simulink model "Plantilla_Simulink_Estanque"  (Simulink 8.1)
settings: Solver=ode5  StartTime=0.0  StopTime=5000  FixedStep=0.05  RelTol=1e-3
libraries: RT x1
settings Model: Creator=Alleon  LastModifiedBy=Admin
settings DataIOCC: LimitDataPoints=off  SaveOutput=off  SaveTime=off  SignalLoggingName=sigsOut
settings OptimizationCC: ExpressionDepthLimit=128  InitFltsAndDblsToZero=on
settings DebuggingCC: SaveWithParameterizedLinksMsg=none  SignalResolutionControl=TryResolveAllWithWarning  SolverPrmCheckMsg=none  MultiTaskDSMMsg=warning  MultiTaskCondExecSysMsg=none  StrictBusMsg=None
settings HardwareCC: TargetUnknown=on
settings SFSimCC: SimParseCustomCode=off
settings RTWCC: IncludeERTFirstTime=on
settings GRTTargetCC: TargetFcnLib=ansi_tfl_tmw.mat

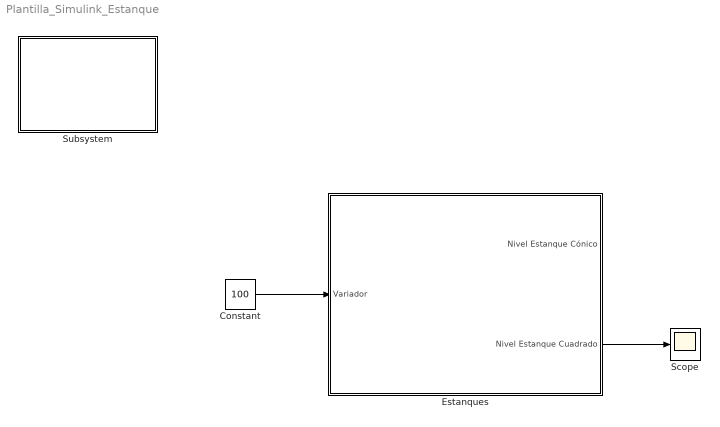
== system Plantilla_Simulink_Estanque ==
  Constant : Constant  Value=100
  Estanques : Subsystem  mask{D=off}
      mask prompts: D "Descarga"
      mask Display:
      | image(imread('img/estanque.png'))
      | 
      | port_label('input', 1, 'Variador')
      | port_label('output', 1, 'Nivel Estanque Conico')
      | port_label('output', 2, 'Nivel Estanque Cuadrado')
  Scope : Scope
      settings: TimeRange=5000  YMin=0  YMax=8.5
  Subsystem : Subsystem
      mask Display: image(imread('img/logo.png'))
  wires:
  Constant/1 -> Estanques/1("Variador ")
  Estanques/2("Nivel Estanque Cuadrado ") -> Scope/1

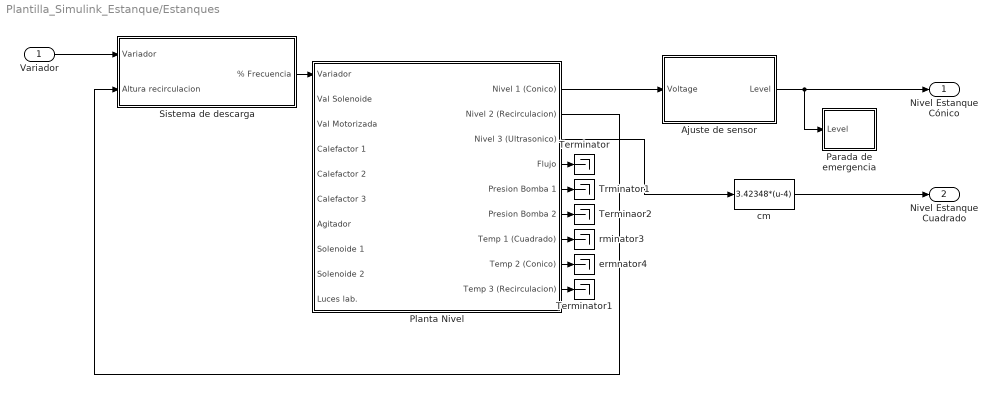
== system Plantilla_Simulink_Estanque/Estanques ==
  "Variador " : Inport
  Ajuste de sensor : Subsystem  mask(Ajuste de sensor){SE=6.53, SL=-0.1}
      mask prompts: SE "Correccion error de sensor"; SL "Limite inferior sensor"
      mask help: Calibra el sensor y transforma la señal de corriente en altura en cms.
  Parada de emergencia : Subsystem  mask(Parada de Emergencia){ML=65}
      mask prompts: ML "Umbral maximo altura"
      mask help: Define el umbral de altura para activar la parada de emergencia.
  Planta Nivel : Subsystem  mask{Ts=0.05}
      mask prompts: Ts "Tiempo Muestreo"
      mask help: Planta de Nivel
  Sistema de descarga : Subsystem  mask{SA=5.28, OT=0.25}
      mask prompts: SA "Ajuste de sensor"; OT "Umbral de apagado"
  Terminaor2 : Terminator
  Terminator : Terminator
  Terminator1 : Terminator
  Trminator1 : Terminator
  cm : Fcn  Expr=3.42348*(u-4)
  ermnator4 : Terminator
  rminator3 : Terminator
  Nivel Estanque Cónico : Outport
  "Nivel Estanque Cuadrado " : Outport  Port=2
  wires:
  Planta Nivel/1(Nivel 1 (Conico)) -> Ajuste de sensor/1(Voltage)
  Planta Nivel/3(Nivel 3 (Ultrasonico)) -> cm/1
  cm/1 -> "Nivel Estanque Cuadrado "/1
  "Variador "/1 -> Sistema de descarga/1(Variador)
  Ajuste de sensor/1(Level) -> Nivel Estanque Cónico/1, Parada de emergencia/1(Level)
  Planta Nivel/2(Nivel 2 (Recirculacion)) -> Sistema de descarga/2(Altura recirculacion)
  Sistema de descarga/1(% Frecuencia) -> Planta Nivel/1(Variador)
  Planta Nivel/4(Flujo) -> Terminator/1
  Planta Nivel/5(Presion Bomba 1) -> Trminator1/1
  Planta Nivel/6(Presion Bomba 2) -> Terminaor2/1
  Planta Nivel/7(Temp 1 (Cuadrado)) -> rminator3/1
  Planta Nivel/8(Temp 2 (Conico)) -> ermnator4/1
  Planta Nivel/9(Temp 3 (Recirculacion)) -> Terminator1/1

== system Plantilla_Simulink_Estanque/Subsystem ==

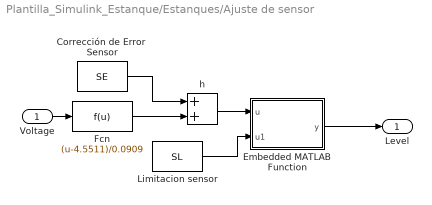
== system Plantilla_Simulink_Estanque/Estanques/Ajuste de sensor ==
  Voltage : Inport
  Corrección de Error  Sensor : Constant  Value=SE  SampleTime=0.05
  Embedded MATLAB Function : MATLAB Function  TreatAsAtomicUnit=on
  Fcn : Fcn  Expr=(u-4.5511)/0.0909
  Limitacion sensor : Constant  Value=SL  SampleTime=0.05
  h : Sum  SampleTime=0.05
  Level : Outport
  wires:
  Corrección de Error  Sensor/1 -> h/1
  h/1 -> Embedded MATLAB Function/1(u)
  Fcn/1 -> h/2
  Embedded MATLAB Function/1(y) -> Level/1
  Voltage/1 -> Fcn/1
  Limitacion sensor/1 -> Embedded MATLAB Function/2(u1)

== system Plantilla_Simulink_Estanque/Estanques/Parada de emergencia ==
  Level : Inport
  Logic : MATLAB Function  TreatAsAtomicUnit=on
  Max. Thres. : Constant  Value=ML
  Stop Simulation : Stop
  wires:
  Logic/1(y) -> Stop Simulation/1
  Level/1 -> Logic/1(u)
  Max. Thres./1 -> Logic/2(u1)

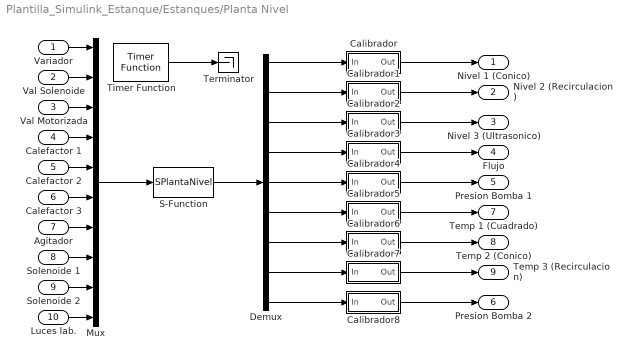
== system Plantilla_Simulink_Estanque/Estanques/Planta Nivel ==
  Variador : Inport
  Val Solenoide : Inport  Port=2
  Val Motorizada : Inport  Port=3
  Calefactor 1 : Inport  Port=4
  Calefactor 2 : Inport  Port=5
  Calefactor 3 : Inport  Port=6
  Agitador : Inport  Port=7
  Solenoide 1 : Inport  Port=8
  Solenoide 2 : Inport  Port=9
  Luces lab. : Inport  Port=10
  Calibrador : Subsystem
  Calibrador1 : Subsystem
  Calibrador2 : Subsystem
  Calibrador3 : Subsystem
  Calibrador4 : Subsystem
  Calibrador5 : Subsystem
  Calibrador6 : Subsystem
  Calibrador7 : Subsystem
  Calibrador8 : Subsystem
  Demux : Demux  Outputs=9
  Mux : Mux  Inputs=10
  S-Function : S-Function  FunctionName=SPlantaNivel  Parameters=Ts  EnableBusSupport=off
  Terminator : Terminator
  Timer Function : RT/Timer Function  Priority=584230560  step=1000*Ts  TaskPriority=NORMAL  ThPriority=TIME CRITICAL
  Nivel 1 (Conico) : Outport
  Nivel 2 (Recirculacion) : Outport  Port=2
  Nivel 3 (Ultrasonico) : Outport  Port=3
  Flujo : Outport  Port=4
  Presion Bomba 1 : Outport  Port=5
  Presion Bomba 2 : Outport  Port=6
  Temp 1 (Cuadrado) : Outport  Port=7
  Temp 2 (Conico) : Outport  Port=8
  Temp 3 (Recirculacion) : Outport  Port=9
  wires:
  Calibrador8/1(Out) -> Presion Bomba 2/1
  Calibrador7/1(Out) -> Temp 3 (Recirculacion)/1
  Calibrador6/1(Out) -> Temp 2 (Conico)/1
  Calibrador5/1(Out) -> Temp 1 (Cuadrado)/1
  Calibrador4/1(Out) -> Presion Bomba 1/1
  Demux/9 -> Calibrador8/1(In)
  Solenoide 2/1 -> Mux/9
  Solenoide 1/1 -> Mux/8
  Calibrador3/1(Out) -> Flujo/1
  Calibrador2/1(Out) -> Nivel 3 (Ultrasonico)/1
  Calibrador1/1(Out) -> Nivel 2 (Recirculacion)/1
  Calibrador/1(Out) -> Nivel 1 (Conico)/1
  Demux/8 -> Calibrador7/1(In)
  Agitador/1 -> Mux/7
  Demux/7 -> Calibrador6/1(In)
  Calefactor 3/1 -> Mux/6
  Demux/6 -> Calibrador5/1(In)
  Calefactor 2/1 -> Mux/5
  Demux/5 -> Calibrador4/1(In)
  Calefactor 1/1 -> Mux/4
  Demux/4 -> Calibrador3/1(In)
  Val Motorizada/1 -> Mux/3
  Demux/3 -> Calibrador2/1(In)
  Val Solenoide/1 -> Mux/2
  Demux/2 -> Calibrador1/1(In)
  Variador/1 -> Mux/1
  Demux/1 -> Calibrador/1(In)
  Mux/1 -> S-Function/1
  S-Function/1 -> Demux/1
  Timer Function/1 -> Terminator/1
  Luces lab./1 -> Mux/10

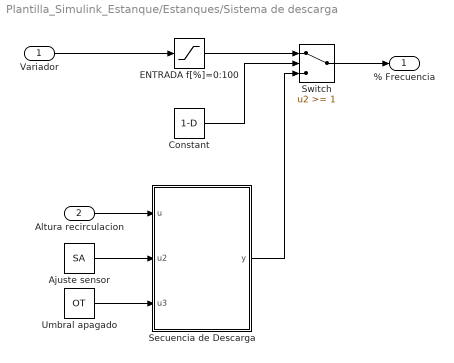
== system Plantilla_Simulink_Estanque/Estanques/Sistema de descarga ==
  Variador : Inport
  Altura recirculacion : Inport  Port=2
  Ajuste sensor : Constant  Value=SA
  Constant : Constant  Value=1-D
  ENTRADA f[%]=0:100 : Saturate  UpperLimit=100  LowerLimit=0  SampleTime=0.05
  Secuencia de Descarga : MATLAB Function  TreatAsAtomicUnit=on
  Switch : Switch  Threshold=1
  Umbral apagado : Constant  Value=OT
  % Frecuencia : Outport
  wires:
  ENTRADA f[%]=0:100/1 -> Switch/1
  Secuencia de Descarga/1(y) -> Switch/3
  Constant/1 -> Switch/2
  Ajuste sensor/1 -> Secuencia de Descarga/2(u2)
  Umbral apagado/1 -> Secuencia de Descarga/3(u3)
  Variador/1 -> ENTRADA f[%]=0:100/1
  Switch/1 -> % Frecuencia/1
  Altura recirculacion/1 -> Secuencia de Descarga/1(u)

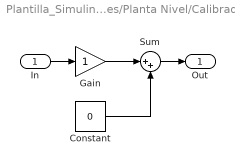
== system Plantilla_Simulink_Estanque/Estanques/Planta Nivel/Calibrador ==
  In : Inport
  Constant : Constant  Value=0
  Gain : Gain  SaturateOnIntegerOverflow=on  OutDataTypeStr=Inherit: Same as input  ParamDataTypeStr=Inherit: Same as input
  Sum : Sum  Inputs=|++  SaturateOnIntegerOverflow=on
  Out : Outport
  wires:
  Sum/1 -> Out/1
  In/1 -> Gain/1
  Constant/1 -> Sum/2
  Gain/1 -> Sum/1

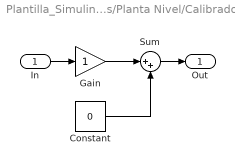
== system Plantilla_Simulink_Estanque/Estanques/Planta Nivel/Calibrador1 ==
  In : Inport
  Constant : Constant  Value=0
  Gain : Gain  SaturateOnIntegerOverflow=on  OutDataTypeStr=Inherit: Same as input  ParamDataTypeStr=Inherit: Same as input
  Sum : Sum  Inputs=|++  SaturateOnIntegerOverflow=on
  Out : Outport
  wires:
  Gain/1 -> Sum/1
  Constant/1 -> Sum/2
  In/1 -> Gain/1
  Sum/1 -> Out/1

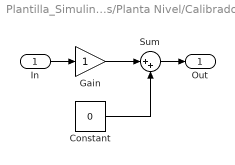
== system Plantilla_Simulink_Estanque/Estanques/Planta Nivel/Calibrador2 ==
  In : Inport
  Constant : Constant  Value=0
  Gain : Gain  SaturateOnIntegerOverflow=on  OutDataTypeStr=Inherit: Same as input  ParamDataTypeStr=Inherit: Same as input
  Sum : Sum  Inputs=|++  SaturateOnIntegerOverflow=on
  Out : Outport
  wires:
  Sum/1 -> Out/1
  In/1 -> Gain/1
  Constant/1 -> Sum/2
  Gain/1 -> Sum/1

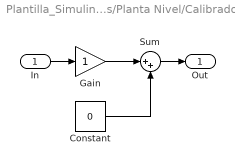
== system Plantilla_Simulink_Estanque/Estanques/Planta Nivel/Calibrador3 ==
  In : Inport
  Constant : Constant  Value=0
  Gain : Gain  SaturateOnIntegerOverflow=on  OutDataTypeStr=Inherit: Same as input  ParamDataTypeStr=Inherit: Same as input
  Sum : Sum  Inputs=|++  SaturateOnIntegerOverflow=on
  Out : Outport
  wires:
  Gain/1 -> Sum/1
  Constant/1 -> Sum/2
  In/1 -> Gain/1
  Sum/1 -> Out/1

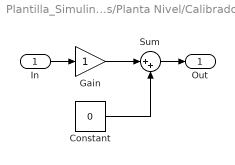
== system Plantilla_Simulink_Estanque/Estanques/Planta Nivel/Calibrador4 ==
  In : Inport
  Constant : Constant  Value=0
  Gain : Gain  SaturateOnIntegerOverflow=on  OutDataTypeStr=Inherit: Same as input  ParamDataTypeStr=Inherit: Same as input
  Sum : Sum  Inputs=|++  SaturateOnIntegerOverflow=on
  Out : Outport
  wires:
  Sum/1 -> Out/1
  In/1 -> Gain/1
  Constant/1 -> Sum/2
  Gain/1 -> Sum/1

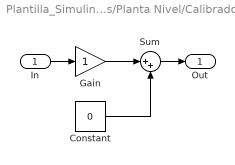
== system Plantilla_Simulink_Estanque/Estanques/Planta Nivel/Calibrador5 ==
  In : Inport
  Constant : Constant  Value=0
  Gain : Gain  SaturateOnIntegerOverflow=on  OutDataTypeStr=Inherit: Same as input  ParamDataTypeStr=Inherit: Same as input
  Sum : Sum  Inputs=|++  SaturateOnIntegerOverflow=on
  Out : Outport
  wires:
  Gain/1 -> Sum/1
  Constant/1 -> Sum/2
  In/1 -> Gain/1
  Sum/1 -> Out/1

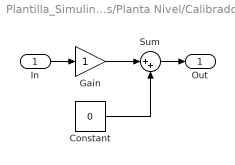
== system Plantilla_Simulink_Estanque/Estanques/Planta Nivel/Calibrador6 ==
  In : Inport
  Constant : Constant  Value=0
  Gain : Gain  SaturateOnIntegerOverflow=on  OutDataTypeStr=Inherit: Same as input  ParamDataTypeStr=Inherit: Same as input
  Sum : Sum  Inputs=|++  SaturateOnIntegerOverflow=on
  Out : Outport
  wires:
  Sum/1 -> Out/1
  In/1 -> Gain/1
  Constant/1 -> Sum/2
  Gain/1 -> Sum/1

== system Plantilla_Simulink_Estanque/Estanques/Planta Nivel/Calibrador7 ==
  In : Inport
  Constant : Constant  Value=0
  Gain : Gain  SaturateOnIntegerOverflow=on  OutDataTypeStr=Inherit: Same as input  ParamDataTypeStr=Inherit: Same as input
  Sum : Sum  Inputs=|++  SaturateOnIntegerOverflow=on
  Out : Outport
  wires:
  Gain/1 -> Sum/1
  Constant/1 -> Sum/2
  In/1 -> Gain/1
  Sum/1 -> Out/1

== system Plantilla_Simulink_Estanque/Estanques/Planta Nivel/Calibrador8 ==
  In : Inport
  Constant : Constant  Value=0
  Gain : Gain  SaturateOnIntegerOverflow=on  OutDataTypeStr=Inherit: Same as input  ParamDataTypeStr=Inherit: Same as input
  Sum : Sum  Inputs=|++  SaturateOnIntegerOverflow=on
  Out : Outport
  wires:
  Sum/1 -> Out/1
  In/1 -> Gain/1
  Constant/1 -> Sum/2
  Gain/1 -> Sum/1

== matlab function Estanques/Sistema de descarga/Secuencia de Descarga ==
  data: u input double; y output double; u2 input double; u3 input double
function y = fcn(u,u2,u3)
% This block supports an embeddable subset of the MATLAB language.
% See the help menu for details. 
u=u-u2;
if u>u3
    y=100;
else
    y=0;
end

== matlab function Estanques/Ajuste de sensor/Embedded MATLAB Function ==
  data: u input double; y output double; u1 input double
function y = fcn(u,u1)
% This block supports an embeddable subset of the MATLAB language.
% See the help menu for details. 
if u <u1
    y=0;
else
y = u;
end

== matlab function Estanques/Parada de emergencia/Logic ==
  data: u input double; y output double; u1 input double
function y = fcn(u,u1)
% This block supports an embeddable subset of the MATLAB language.
% See the help menu for details. 
if u>=u1
    y=1;
else
    y=0;
end
